simulink model "Force_Control_05_10_23"  (R2023a)
settings: Solver=VariableStepAuto  StartTime=0.0  StopTime=40  RelTol=1e-3
values from neighbouring files (symbols this model uses):
  N = [-y1+y3;-x3+x1]    [Contact.m]
  X = 0.65    [Contact.m]    (also in FFFB_PosForce_ME.m = [X0',X1',X2']; FFFB_PosForce_ME1.m = [X2']; FFFB_PosForce_ME2.m = [X110,X2']; FFFB_Posarbitary_actual_Mass.m = [X110])
  Y = [Y0',Y1',Y2']    [FFFB_PosForce_ME.m]    (also in FFFB_PosForce_ME1.m = [Y2']; FFFB_PosForce_ME2.m = [Y110,Y2']; FFFB_Posarbitary_actual_Mass.m = [Y110]; FFFB_arbitary_actual_Mass.m = [Y2'])
undefined symbols (not defined in the file or in its folder): Z
libraries: sm_lib x44, nesl_utility x14
(part 2 of 2)

== matlab function Force_Control_05_10_23/MATLAB Function2 ==
  data: q1 input; PP output; q2 input
function PP = fcn(q1,q2)
phi1=-1.57;
a1_=0.0001;
b1_=0.0001;
a1=0.05;
a2=0.05;
L01=0.05;
PP=R_EQ(L01,a1,a2,a1_,b1_,phi1,q1,q2);

== matlab function Force_Control_05_10_23/Desired2 ==
  data: PP output; t input; Pdd output; Fd output
function [PP,Pdd,Fd]=fun1(t)

Yf=0.02;
Xf0=0.05-0.01+0.025;
Xfs=Xf0+0.02;
Xf0_d=0;
Xf0_dd=0;
ts=40;
[Xf,Xf_d,Xf_dd]=para_(Xf0,Xf0_d,Xf0_dd,t,ts,Xfs);
PP=[Xf;Yf];
Pd=[Xf_d;0];
Pdd=[Xf_dd;0];
Fd=[0.010;001]

== matlab function Force_Control_05_10_23/MATLAB Function ==
  data: u input; y output
function y = fcn(u)

Jac = R_Jac1(a1,a2,a1_,b1_,phi1,q1,q2);
Jd=R_Jd1(a1,a2,a1_,b1_,phi1,q1,q2,q1dot,q2dot);
Fd=[0.1];
aq11=aq1;
aq21=aq2;
% end
M=R_M(C1,C2,Itot1(9),Itot2(9),a1,m1,m2+m3,q2);
C =  R_damp(C2,a1,m2+m3,q2,q1dot,q2dot);
G= R_Gra(C1,C2,a1,m1,m2+m3,g,q1,q2);
M_=inv(Jac')*M*inv(Jac);
nt=inv(Jac')*(-M*inv(Jac)*Jd*[q1dot;q1dot]+(C+G));
A = [0,1];
x1=1;

P=eye(2)-(A'*inv(A*inv(M_)*A')*A*inv(M_))*x1;
F1=P*(M_*[aq1;aq2]+nt);
F2=(eye(2)-P)*(M_*[aq11;aq21]+nt+A'*Fd);
F=F1+F2;
F11=[F1 F2 F]
u =Jac'*(P*(M_*[aq1;aq2]+nt));
DD=inv(Jac')*(inv(P*M_)*(P*nt))

== matlab function Force_Control_05_10_23/Inner Loop Control1 ==
  data: q1 input; u1 output; q2 input; q1dot input; q2dot input; aq1 input; aq2 input; u2 output; u1_ output; u2_ output
function [u1,u2,u1_,u2_] = fcn(q1,q2,q1dot,q2dot,aq1,aq2)
g=9.81;
a1=0.05;  
a2=0.05; 
L01=0.05;
m1=0.00156;
m2=0.00156;
m3=4.90088e-05;
a1_=0.001;
b1_=0.001;
phi1=-0.8;
% m3=0;
C1=a1/2;
C2=(m2*0.5*a2+m3*a2)/(m2+m3);

r=0.001;
I1=[0 0 0;0 m1*a1^2/12 0;0 0 m1*a1^2/12];
I2=[0 0 0;0 m2*a2^2/12 0;0 0 m2*a2^2/12];
I3=[0 0 0;0 m3*r^2/2 0;0 0 m3*r^2/2];

Itot1=I1; 
Itot2=I2+I3+[zeros(2,3);zeros(1,2) m3*(C2-a2)^2]; 
Jac = R_Jac(a1,a2,q1,q2)
Jd=R_Jd(a1,a2,q1,q2,q1dot,q2dot);
M=R_M(C1,C2,Itot1(9),Itot2(9),a1,m1,m2+m3,q2);
C =  R_damp(C2,a1,m2+m3,q2,q1dot,q2dot);
G= R_Gra(C1,C2,a1,m1,m2+m3,g,q1,q2);

u = M*inv(Jac)*[aq1;aq2]-M*inv(Jac)*Jd*[q1dot;q2dot]+C+G;

u1=u(1);
u2=u(2);

M_=inv(Jac')*M*inv(Jac);
nt=inv(Jac')*(-M*inv(Jac)*Jd*[q1dot;q1dot]+(C+G));
A=[0,1];
P=eye(2)-(A'*inv(A*inv(M_)*A')*A*inv(M_));
u_ =Jac'*P*(M_*[aq1;aq2]+nt);
u1_=u_(1);
u2_=u_(2);

== matlab function Force_Control_05_10_23/MATLAB Function1 ==
  data: q1 input; PP output; q2 input
function PP = fcn(q1,q2)
phi1=-1.57;
a1_=0.0001;
b1_=0.0001;
a1=0.05;
a2=0.05;
L01=0.05;
PP=R_EQ(L01,a1,a2,a1_,b1_,phi1,q1,q2);

== matlab function Force_Control_05_10_23/Inner Loop Control3 ==
  data: q1 input; DD1 output; q2 input; q1dot input; q2dot input; aq1 input; aq2 input; DD2 output; Fd input; aq11 input; aq21 input
function [DD1,DD2] =  fcn(q1,q2,q1dot,q2dot,aq1,aq2,Fd,aq11,aq21)
g=9.81;
a1=0.05;  
a2=0.05; 
L01=0.05;
m1=0.00156;
m2=0.00156;
m3=4.90088e-05;
a1_=0.001;
b1_=0.001;
phi1=-1.57;
% m3=0;
C1=a1/2;
C2=(m2*0.5*a2+m3*a2)/(m2+m3);

r=0.001;
I1=[0 0 0;0 m1*a1^2/12 0;0 0 m1*a1^2/12];
I2=[0 0 0;0 m2*a2^2/12 0;0 0 m2*a2^2/12];
I3=[0 0 0;0 m3*r^2/2 0;0 0 m3*r^2/2];

Itot1=I1; 
Itot2=I2+I3+[zeros(2,3);zeros(1,2) m3*(C2-a2)^2]; 
% if t<=40
Jac = R_Jac1(a1,a2,a1_,b1_,phi1,q1,q2);
Jd=R_Jd1(a1,a2,a1_,b1_,phi1,q1,q2,q1dot,q2dot);

% end
M=R_M(C1,C2,Itot1(9),Itot2(9),a1,m1,m2+m3,q2);
C =  R_damp(C2,a1,m2+m3,q2,q1dot,q2dot);
G= R_Gra(C1,C2,a1,m1,m2+m3,g,q1,q2);
M_=inv(Jac')*M*inv(Jac);
nt=inv(Jac')*(-M*inv(Jac)*Jd*[q1dot;q1dot]+(C+G));
A = [0 0;0 1];
P=eye(2)-(A'*inv(A*inv(M_)*A')*A*inv(M_));
u =Jac'*(P*(M_*[aq1;aq2]+nt)+(eye(2)-P)*(nt+A'*Fd));
DD=inv(M)*(u-C-G-Jac'*A'*Fd);
DD1=DD(1);
DD2=DD(2);

== matlab function Force_Control_05_10_23/Desired1 ==
  data: PP output; t input; Pdd output; Fd output
function [PP,Pdd,Fd]=fun1(t)

Yf=0.02;
Xf0=0.05-0.01+0.025;
Xfs=Xf0+0.02;
Xf0_d=0;
Xf0_dd=0;
ts=40;
[Xf,Xf_d,Xf_dd]=para_(Xf0,Xf0_d,Xf0_dd,t,ts,Xfs);
PP=[Xf;Yf];
Pd=[Xf_d;0];
Pdd=[Xf_dd;0];
Fd=[0;0]

== matlab function Force_Control_05_10_23/Inner Loop Control2 ==
  data: q1 input; DD1 output; q2 input; q1dot input; q2dot input; aq1 input; aq2 input; DD2 output; Fd input; aq11 input; aq21 input
function [DD1,DD2] =  fcn(q1,q2,q1dot,q2dot,aq1,aq2,Fd,aq11,aq21)
g=9.81;
a1=0.05;  
a2=0.05; 
L01=0.05;
m1=0.00156;
m2=0.00156;
m3=4.90088e-05;
a1_=0.001;
b1_=0.001;
phi1=-1.57;
% m3=0;
C1=a1/2;
C2=(m2*0.5*a2+m3*a2)/(m2+m3);

r=0.001;
I1=[0 0 0;0 m1*a1^2/12 0;0 0 m1*a1^2/12];
I2=[0 0 0;0 m2*a2^2/12 0;0 0 m2*a2^2/12];
I3=[0 0 0;0 m3*r^2/2 0;0 0 m3*r^2/2];

Itot1=I1; 
Itot2=I2+I3+[zeros(2,3);zeros(1,2) m3*(C2-a2)^2]; 
% if t<=40
Jac = R_Jac1(a1,a2,a1_,b1_,phi1,q1,q2);
Jd=R_Jd1(a1,a2,a1_,b1_,phi1,q1,q2,q1dot,q2dot);

% end
M=R_M(C1,C2,Itot1(9),Itot2(9),a1,m1,m2+m3,q2);
C =  R_damp(C2,a1,m2+m3,q2,q1dot,q2dot);
G= R_Gra(C1,C2,a1,m1,m2+m3,g,q1,q2);
M_=inv(Jac')*M*inv(Jac);
nt=inv(Jac')*(-M*inv(Jac)*Jd*[q1dot;q1dot]+(C+G));
A = [0 0;0 1];
P=eye(2)-(A'*inv(A*inv(M_)*A')*A*inv(M_));
u =Jac'*(P*(M_*[aq1;aq2]+nt)+(eye(2)-P)*(nt+A'*Fd));
DD=inv(M)*(u-C-G-Jac'*A'*Fd);
DD1=DD(1);
DD2=DD(2);
